simulink model "System_model"  (R2024b)
settings: Solver=FixedStepAuto  StartTime=0.0  StopTime=24*60  FixedStep=1  RelTol=1e-3
undefined symbols (not defined in the file): A, c, E_boiler_0, E_load_0, E_request_0, E_solar_0, epsilon, eta_zero, I_timeseries, m_dot, mu_timeseries, Ta_timeseries, tank_loss_coeff, Tank_volume, Thome, Tin_0, Tmains, Ts0, Tu_timeseries, U
settings Model: Creator=giacm  LastModifiedBy=Andrea
settings RTWCC: GPUComputeCapability=3.5

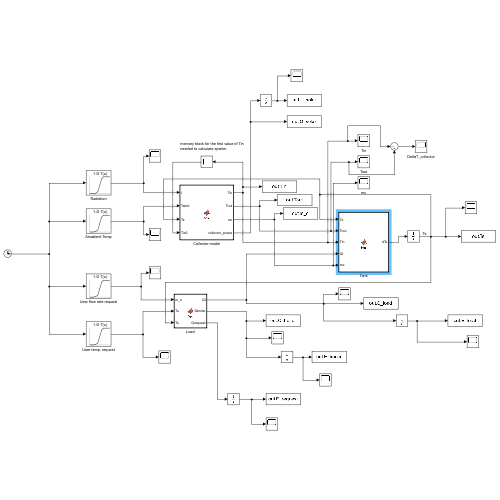
[thumbnail: Simulink's stored preview of the top-level diagram]
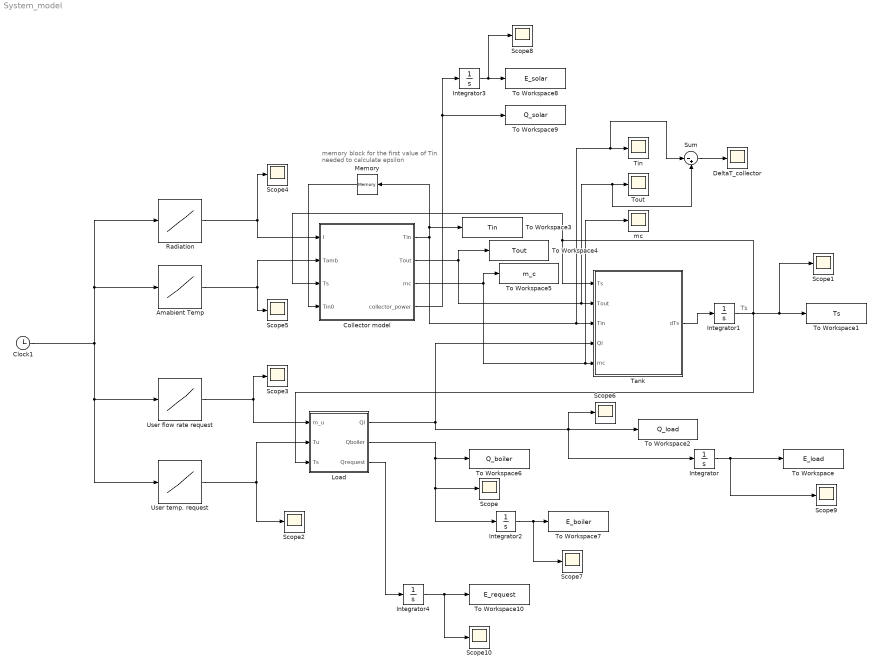
== system System_model ==
  note: memory block for the first value of Tin
      | needed to calculate epsilon
  note: Ts
  Amabient Temp : Lookup_n-D  NumberOfTableDimensions=1  BreakpointsForDimension1=Ta_timeseries.Time  Table=Ta_timeseries.Data  InternalRulePriority=Speed  RndMeth=Simplest
  Clock1 : Clock
  Collector model : MATLAB Function  TreatAsAtomicUnit=on
  DeltaT_collector : Scope
  Integrator : Integrator  InitialCondition=E_load_0
  Integrator1 : Integrator  InitialCondition=Ts0
  Integrator2 : Integrator  InitialCondition=E_boiler_0
  Integrator3 : Integrator  InitialCondition=E_solar_0
  Integrator4 : Integrator  InitialCondition=E_request_0
  Load : MATLAB Function  TreatAsAtomicUnit=on
  Memory : Memory  InitialCondition=Tin_0
  Radiation : Lookup_n-D  NumberOfTableDimensions=1  BreakpointsForDimension1=I_timeseries.Time  Table=I_timeseries.Data  InternalRulePriority=Speed  RndMeth=Simplest
  Scope{,1..10} (11 alike) : Scope
  Sum : Sum  Inputs=|-+
  Tank : MATLAB Function  TreatAsAtomicUnit=on
  Tin : Scope
  To Workspace : ToWorkspace  VariableName=E_load  SampleTime=-1
  To Workspace1 : ToWorkspace  VariableName=Ts  SampleTime=-1
  To Workspace10 : ToWorkspace  VariableName=E_request  SampleTime=-1
  To Workspace2 : ToWorkspace  VariableName=Q_load  SampleTime=-1
  To Workspace3 : ToWorkspace  VariableName=Tin  SampleTime=-1
  To Workspace4 : ToWorkspace  VariableName=Tout  SampleTime=-1
  To Workspace5 : ToWorkspace  VariableName=m_c  SampleTime=-1
  To Workspace6 : ToWorkspace  VariableName=Q_boiler  SampleTime=-1
  To Workspace7 : ToWorkspace  VariableName=E_boiler  SampleTime=-1
  To Workspace8 : ToWorkspace  VariableName=E_solar  SampleTime=-1
  To Workspace9 : ToWorkspace  VariableName=Q_solar  SampleTime=-1
  Tout : Scope
  User flow rate request : Lookup_n-D  NumberOfTableDimensions=1  BreakpointsForDimension1=mu_timeseries.Time  Table=mu_timeseries.Data  InternalRulePriority=Speed  RndMeth=Simplest
  User temp. request : Lookup_n-D  NumberOfTableDimensions=1  BreakpointsForDimension1=Tu_timeseries.Time  Table=Tu_timeseries.Data  InternalRulePriority=Speed  RndMeth=Simplest
  mc : Scope
  wires:
  Clock1/1 -> User flow rate request/1, User temp. request/1, Amabient Temp/1, Radiation/1
  Collector model/1(Tin) -> Sum/1, Tin/1, Tank/3(Tin), To Workspace3/1, Memory/1
  Amabient Temp/1 -> Collector model/2(Tamb), Scope5/1
  Radiation/1 -> Collector model/1(I), Scope4/1
  User flow rate request/1 -> Scope3/1, Load/1(m_u)
  User temp. request/1 -> Scope2/1, Load/2(Tu)
  Collector model/3(mc) -> mc/1, Tank/5(mc), To Workspace5/1
  Collector model/2(Tout) -> Tout/1, Sum/2, Tank/2(Tout), To Workspace4/1
  Load/1(Ql) -> Integrator/1, To Workspace2/1, Scope6/1, Tank/4(Ql)
  Load/2(Qboiler) -> To Workspace6/1, Scope/1, Integrator2/1
  Tank/1(dTs) -> Integrator1/1
  Integrator1/1 -> Scope1/1, To Workspace1/1, Tank/1(Ts), Collector model/3(Ts), Load/3(Ts)
  Memory/1 -> Collector model/4(Tin0)
  Sum/1 -> DeltaT_collector/1
  Integrator2/1 -> Scope7/1, To Workspace7/1
  Integrator3/1 -> Scope8/1, To Workspace8/1
  Collector model/4(collector_power) -> To Workspace9/1, Integrator3/1
  Integrator/1 -> Scope9/1, To Workspace/1
  Integrator4/1 -> Scope10/1, To Workspace10/1
  Load/3(Qrequest) -> Integrator4/1

== matlab function System_model/Collector model ==
  data: I input; Tamb input; Ts input; Tin output; Tout output; mc output; Tin0 input; eta_zero parameter; U parameter; m_dot parameter; A parameter; c parameter; epsilon parameter; collector_power output
function [Tin, Tout, mc, collector_power] = fcn(I,Tamb,Ts, Tin0, eta_zero, U, m_dot, A, c, epsilon)


%to add: starting from a set Tin, find a way to make eta calculate itself
eta = eta_zero - (U * ((Tin0 - Tamb) / I));

% Open valve only if we have irradiation and positive eta. Assume constant
% flow rate if valve is open (given by producer)

if(I > 0 && eta > 0)
    mc = m_dot;
else
    mc = 0;
end


if(isnan(eta) || isinf(eta))
    collector_power = 0;
else
    collector_power = eta * I * A;     % [W]
end

%wrong
%deltaT_collector = collector_power / (mc * c_joule)
%Tout = Tin + deltaT_collector;


%from Maple
% check if it is NaN (0/0)
temp1 = (mc * c * epsilon * (Ts + 273.15) + collector_power) / (mc * c * epsilon);      % [K] in Kelvin because of c

if (isnan(temp1) || isinf(temp1))
    % we should model this with a heat loss coefficient (when mc=0), however it doesn't quite
    % matter because when mc is zero Tout has no effect on Ts (see tank
    % block). As soon as the collector pump starts working we compute the
    % actual value of Tout.
    Tout = Ts;
else
    Tout = (temp1 - 273.15);    % [C] Celsius
end

Tin = Tout - epsilon * (Tout - Ts);

== matlab function System_model/Tank ==
  data: dTs output; Ts input; Tout input; Tin input; Ql input; mc input; tank_loss_coeff parameter; A parameter; Thome parameter; c parameter; Tank_volume parameter
function dTs = fcn(Ts, Tout, Tin, Ql, mc, tank_loss_coeff, A, Thome, c, Tank_volume)

Qloss = tank_loss_coeff*A*(Ts-Thome);
%Qloss = 0;

sos = (mc*c*(Tout-Tin) - Ql - Qloss) / (Tank_volume * c);   % This should be in Kelvin but i guess it's fine because after all it's a derivative (so a kind of deltaT)

if (isnan(sos) || isinf(sos))
    dTs = 0;
else
    dTs = sos;
end

== matlab function System_model/Load ==
  data: m_u input; Ql output; Tu input; Ts input; Qboiler output; c parameter; Tmains parameter; Qrequest output
function [Ql, Qboiler, Qrequest] = fcn(m_u, Tu, Ts, c, Tmains)

if(Tu <= Ts)
    Ql = m_u * c * (Tu - Tmains);
else
    Ql = m_u * c * (Ts - Tmains);
end

if(Tu <= Ts)
    Qboiler = 0;
else
    Qboiler = m_u * c * (Tu - Ts);
end


Qrequest = m_u * c * (Tu - Tmains);


end
